simulink model "snap2_f_200msps_64i_4096c"  (R2019a)
settings: Solver=VariableStepDiscrete  StartTime=0.0  StopTime=10.0  RelTol=1e-3
undefined symbols (not defined in the file or in its folder): datetime, posixtime
libraries: xbsIndex_r4 x21354, casper_library_misc x297, casper_library_delays x19, xps_library x14, casper_library_sources x4
(part 1 of 217)
settings Model: ModifiedComment=jackh -- Fri May 23 06:17:14 2025 -- Version 1.665  Creator=mdexter  LastModifiedBy=jackh
settings Model: ModifiedHistory=|
  | jackh -- Fri May 23 06:17:14 2025 -- Version 1.665
  | 
  | jackh -- Thu May 22 05:48:14 2025 -- Version 1.664
  | 
  | v7.4.0.0 -- Expand number of coefficients to one per channel
  | 
  | kplant -- Fri Aug 11 09:07:04 2023 -- Version 1.663
  | Saving after compiling
  | 
  | kplant -- Thu Aug 10 22:12:33 2023 -- Version 1.662
  | Version 7.3.2.1 now has pipelines with a latency of 3 before the f-engine's ethernet block.
  | 
  | kplant -- Thu Aug 10 10:59:50 2023 -- Version 1.661
  | Version 7.3.2.0 increases the pipeline latency to 2 in front of the f-engine 40Gbe block and changes the target clock rate to 196 MHz.
  | 
  | kplant -- Wed Aug 09 13:06:15 2023 -- Version 1.660
  | Added pipeline blocks with a latency of 1 before each of the inputs to the 40Gb ethernet block that the f-engine uses.
  | 
  | kplant -- Tue Aug 08 14:00:49 2023 -- Version 1.659
  | 
  | kplant -- Tue Aug 08 13:55:20 2023 -- Version 1.658
  | Adding cosmic ray system version 6.0.1.0 which has the FIR and so far has only been compiled from snap2_f_200msps_64i_4096c_nopfb.slx
  | 
  | kplant -- Thu Apr 27 20:02:10 2023 -- Version 1.657
  | Saving after compile.
  | 
  | kplant -- Wed Apr 26 17:00:51 2023 -- Version 1.656
  | I removed the delay trigger option and changed it to an option to delay the input to the buffer, in order to be able to position the pulse in the center of the buffer.
  | 
  | kplant -- Fri Apr 07 12:31:25 2023 -- Version 1.655
  | Add cosmic ray version 5.0.0.1 and change main version to 7.3.0.2.
  | 
  | kplant -- Thu Apr 06 14:32:58 2023 -- Version 1.654
  | Saving after compiling 7.3.0.1.
  | 
  | jackh -- Thu Apr 06 12:53:56 2023 -- Version 1.653
  | 
  | Make CR block and mask block use sync_time, not telescope_time
  | 
  | kplant -- Fri Mar 24 06:24:14 2023 -- Version 1.652
  | Saving after compiling version 7.3 with cosmic ray system 5.0.0.
  | 
  | jackh -- Wed Mar 08 22:10:30 2023 -- Version 1.651
  | 
  | compiled
  | 
  | jackh -- Wed Mar 08 15:15:31 2023 -- Version 1.650
  | rev 7.2
  | 2 bits below EQ binary point
  | 
  | jackh -- Thu Feb 16 17:13:47 2023 -- Version 1.649
  | 
  | compiled
  | 
  | jackh -- Thu Feb 16 09:43:58 2023 -- Version 1.648
  | 
  | Remove hard-coded first 5-stages of shift
  | 
  | jackh -- Wed Feb 15 17:04:22 2023 -- Version 1.647
  | 
  | compiled
  | 
  | jackh -- Tue Feb 14 18:32:23 2023 -- Version 1.646
  | 
  | Change EQ fractional bits from 5 to 4
  | Rebuild FFT IP with all serial stages optional shift
  | 
  | jackh -- Thu Jan 05 10:26:17 2023 -- Version 1.645
  | v7.0.0 as compiled
  | 
  | jackh -- Wed Jan 04 19:36:26 2023 -- Version 1.644
  | 
  | jackh -- Wed Jan 04 19:34:58 2023 -- Version 1.643
  | v7.0.0.0
  | CR version 4.3.1
  | 
  | jackh -- Tue Dec 20 11:37:43 2022 -- Version 1.642
  | 
  | compiled 6.1. 4 x 0.003ns timing errors, only on unused CR 40GbE RX path.
  | 
  | 
  | jackh -- Fri Dec 16 15:06:04 2022 -- Version 1.641
  | 
  | jackh -- Fri Dec 16 14:46:34 2022 -- Version 1.640
  | 
  | jackh -- Fri Dec 16 14:13:03 2022 -- Version 1.639
  | 
  | jackh -- Fri Dec 16 13:41:06 2022 -- Version 1.638
  | 
  | 6.1 -- add per-signal flag threshold
  | 
  | jackh -- Fri Dec 16 11:47:24 2022 -- Version 1.637
  | 
  | jackh -- Fri Dec 16 11:47:00 2022 -- Version 1.636
  | 
  | jackh -- Thu Dec 15 20:54:27 2022 -- Version 1.635
  | 
  | Add acc_time registers
  | 
  | jackh -- Thu Dec 15 12:49:42 2022 -- Version 1.634
  | 
  | Include all 4 mask cores (whoops!)
  | 
  | jackh -- Thu Dec 15 12:39:59 2022 -- Version 1.633
  | 
  | Change max coarse delay to 4096 (previous compile didn't meet timing)
  | 
  | jackh -- Wed Dec 14 18:27:06 2022 -- Version 1.632
  | 
  | Add "mask" block, which allows zero-ing out spectra
  | whose total power exceed a runtime-controllable
  | threshold
  | 
  | kplant -- Wed Jun 01 13:17:05 2022 -- Version 1.631
  | 
  | kplant -- Wed Jun 01 07:18:09 2022 -- Version 1.630
  | 
  | kplant -- Wed Jun 01 06:41:48 2022 -- Version 1.629
  | Fixed telescope time input to cosmic ray block.
  | 
  | kplant -- Wed Jun 01 06:39:11 2022 -- Version 1.628
  | Commented out scopes
  | 
  | kplant -- Tue May 31 12:58:33 2022 -- Version 1.627
  | Cosmic ray version 4.1. Takes in telescope time, attempts to fix bug where trigger signal is blocked from starting packetizer.
  | 
  | kplant -- Tue May 31 12:56:22 2022 -- Version 1.626
  | 
  | kplant -- Tue May 31 09:44:09 2022 -- Version 1.625
  | 
  | jackh -- Fri May 13 14:05:09 2022 -- Version 1.624
  | 
  | Compiled 5.1.1.0 (CR rev 4)
  | 
  | jackh -- Thu May 12 12:01:29 2022 -- Version 1.623
  | 
  | Add PPS count register (which software already assumes exists!)
  | 
  | jackh -- Thu May 12 11:34:03 2022 -- Version 1.622
  | 
  | v5.1.0
  | Manual merge in of v4.0 CR module
  | 
  | jackh -- Thu Apr 14 04:49:04 2022 -- Version 1.621
  | 
  | jackh -- Wed Mar 23 12:35:09 2022 -- Version 1.620
  | 
  | Manually merce cosmic_ray_system.slx into the cosmic_ray subsystem
  | of this model. cosmic_ray_system appears to be version 3 (based on version register).
  | 
  | Bump main model version to 5.0.0.0
  | 
  | jackh -- Tue Jan 11 12:36:06 2022 -- Version 1.619
  | 
  | jackh -- Mon Jan 10 21:45:35 2022 -- Version 1.618
  | 
  | Bump bugfix
  | 
  | jackh -- Mon Jan 10 21:43:35 2022 -- Version 1.617
  | 
  | jackh -- Mon Jan 10 21:39:42 2022 -- Version 1.616
  | 
  | jackh -- Mon Jan 10 21:33:55 2022 -- Version 1.615
  | 
  | jackh -- Mon Jan 10 21:16:30 2022 -- Version 1.614
  | 
  | Fix bit width of sum(sq(ADC value)) -- was configured for 8 bit ADCs!
  | 
  | jackh -- Mon Nov 15 21:56:57 2021 -- Version 1.613
  | 
  | compiled
  | 
  | jackh -- Mon Nov 15 11:54:45 2021 -- Version 1.612
  | 
  | v4.6.0 -- add internal loopback for sync logic
  | 
  | jackh -- Fri Sep 17 19:23:29 2021 -- Version 1.611
  | 
  | Compiled with clean timing
  | 
  | 
  | jackh -- Fri Sep 17 13:13:59 2021 -- Version 1.610
  | 4.5.4 CR update
  | 
  | jackh -- Tue Sep 14 19:01:48 2021 -- Version 1.609
  | 
  | jackh -- Tue Sep 14 10:37:44 2021 -- Version 1.608
  | 
  | Change CR buffer BRAMs to have latency 2 and optimize for speed.
  | 
  | jackh -- Mon Sep 13 20:49:56 2021 -- Version 1.607
  | 
  | jackh -- Mon Sep 13 20:30:25 2021 -- Version 1.606
  | 
  | 4.5.3
  | Increase latency of autocorr vacc adders to 4
  | Change CR veto pulse extend subtract-1 to implement behaviourally
  | 
  | jackh -- Mon Sep 13 20:29:50 2021 -- Version 1.605
  | 
  | jackh -- Mon Sep 13 10:57:29 2021 -- Version 1.604
  | 
  | v4.5.2
  | 
  | Update CR subsys. Not sure whether this has actually changed,
  | but there was a commit to the repo. Using 14655219acb09ca
  | 
  | jackh -- Mon Sep 13 10:51:07 2021 -- Version 1.603
  | 
  | jackh -- Sun Sep 12 12:08:30 2021 -- Version 1.602
  | 
  | 4.5.1 -- update CR subsys
  | 
  | jackh -- Tue Aug 31 13:12:34 2021 -- Version 1.601
  | 
  | jackh -- Wed Aug 25 19:11:33 2021 -- Version 1.600
  | 
  | jackh -- Tue Aug 24 13:10:24 2021 -- Version 1.599
  | 
  | Fix delay readout bug
  | 
  | jackh -- Tue Aug 24 12:10:39 2021 -- Version 1.598
  | 
  | compiled. Missed timing, but only on 40G RX paths and within the 200MHz->196MHz margin
  | 
  | jackh -- Mon Aug 23 18:54:36 2021 -- Version 1.597
  | 
  | update CR
  | 
  | jackh -- Mon Aug 23 18:52:51 2021 -- Version 1.596
  | 
  | compiled
  | 
  | jackh -- Mon Aug 16 15:01:28 2021 -- Version 1.595
  | 
  | re-fix delay readout
  | 
  | jackh -- Mon Aug 16 14:36:11 2021 -- Version 1.594
  | 
  | compiled v4.3.0
  | 
  | jackh -- Fri Aug 13 12:33:00 2021 -- Version 1.593
  | 
  | jackh -- Fri Aug 13 12:32:21 2021 -- Version 1.592
  | 
  | jackh -- Fri Aug 13 12:30:04 2021 -- Version 1.591
  | 
  | Make autocorr vacc all float32
  | 
  | jackh -- Fri Aug 13 12:16:09 2021 -- Version 1.590
  | 
  | jackh -- Fri Aug 13 12:09:57 2021 -- Version 1.589
  | 
  | jackh -- Thu Aug 12 18:59:45 2021 -- Version 1.588
  | 
  | jackh -- Thu Aug 12 10:15:56 2021 -- Version 1.587
  | 
  | Remove CR 40GbE TX snapshot
  | 
  | jackh -- Thu Aug 12 10:13:47 2021 -- Version 1.586
  | 
  | Misc pipelining
  | 
  | jackh -- Wed Aug 11 12:31:06 2021 -- Version 1.585
  | 
  | jackh -- Wed Aug 11 12:26:16 2021 -- Version 1.584
  | 
  | v4.4
  | 
  | jackh -- Wed Aug 11 12:25:20 2021 -- Version 1.583
  | 
  | Combine some software registers in CR subsys
  | Combine delay registers into a RAM to (try to) reduce wishbone interconnect
  | 
  | jackh -- Wed Aug 11 11:56:18 2021 -- Version 1.582
  | 
  | Change delay registering to store delays in bram
  | 
  | jackh -- Wed Aug 11 11:10:53 2021 -- Version 1.581
  | 
  | Reduce number of noise generators to 4.
  | Control noise fanout to multiplexers
  | 
  | jackh -- Tue Aug 10 11:27:32 2021 -- Version 1.580
  | 
  | jackh -- Tue Aug 10 11:26:01 2021 -- Version 1.579
  | 
  | fix EQ coefficient addressing
  | 
  | jackh -- Tue Aug 10 11:02:45 2021 -- Version 1.578
  | 
  | jackh -- Mon Aug 09 21:32:19 2021 -- Version 1.577
  | 
  | jackh -- Mon Aug 09 21:31:35 2021 -- Version 1.576
  | 
  | jackh -- Mon Aug 09 18:30:08 2021 -- Version 1.575
  | 
  | compiled
  | 
  | jackh -- Mon Aug 09 10:43:25 2021 -- Version 1.574
  | 
  | jackh -- Mon Aug 09 10:40:58 2021 -- Version 1.573
  | 
  | jackh -- Mon Aug 09 10:31:43 2021 -- Version 1.572
  | 
  | Add pipeline registers on high-fanout CR subsystem sw register outputs
  | 
  | jackh -- Sun Aug 08 14:34:28 2021 -- Version 1.571
  | 
  | v4.3.0
  | 
  | jackh -- Sun Aug 08 14:24:45 2021 -- Version 1.570
  | 
  | jackh -- Sun Aug 08 14:11:25 2021 -- Version 1.569
  | 
  | jackh -- Sun Aug 08 13:31:26 2021 -- Version 1.568
  | 
  | Go back to floating point autocorr. Previous design used more ram and failed timing
  | 
  | jackh -- Sat Aug 07 15:01:43 2021 -- Version 1.567
  | 
  | Change chan_reorder double buffers to optimize for area
  | (sometimes halves the number of brams)
  | 
  | jackh -- Sat Aug 07 14:54:24 2021 -- Version 1.566
  | 
  | v4.2.0
  | 
  | Make autocorr 64-bit fixed point (to save floating cast)
  | Remove serial reorder from FFT and make part of EQ.
  | Compensate by bitbashing addresses for autocorr readout and EQ coefficients
  | 
  | 
  | jackh -- Sat Aug 07 14:49:26 2021 -- Version 1.565
  | 
  | jackh -- Sat Aug 07 14:41:23 2021 -- Version 1.564
  | 
  | jackh -- Sat Aug 07 14:24:43 2021 -- Version 1.563
  | 
  | jackh -- Sat Aug 07 13:38:58 2021 -- Version 1.562
  | 
  | Try to optimize pre-PFB reorder buffers
  | 
  | jackh -- Sat Aug 07 13:18:16 2021 -- Version 1.561
  | 
  | jackh -- Sat Aug 07 13:16:02 2021 -- Version 1.560
  | 
  | Put back in clip count registers because LRD uses them
  | 
  | jackh -- Sat Aug 07 12:39:11 2021 -- Version 1.559
  | 
  | jackh -- Sat Aug 07 12:19:25 2021 -- Version 1.558
  | 
  | compiled. Missed timing on one path by 0.04ns
  | 
  | jackh -- Tue Aug 03 11:43:54 2021 -- Version 1.557
  | 
  | jackh -- Tue Aug 03 11:14:29 2021 -- Version 1.556
  | 
  | Fix double up of delay RAM
  | 
  | jackh -- Tue Aug 03 11:04:58 2021 -- Version 1.555
  | 
  | 4.2.1 -- put CR QSP on port 2
  | 
  | jackh -- Mon Aug 02 12:46:12 2021 -- Version 1.554
  | 
  | Remove RX-side debug counters in CR 40G core
  | 
  | jackh -- Mon Aug 02 12:36:50 2021 -- Version 1.553
  | 
  | Make input power calculation use DSP
  | Change some input delays to behavioural
  | Change delay block to implement a single delay
  | with programmable delay from 0 to 1023, followed by 7
  | fixed 1024 clock delays which may be optionally bypassed.
  | Hopefully this will use less power.
  | 
  | jackh -- Mon Aug 02 11:15:00 2021 -- Version 1.552
  | 
  | implementation optimizations in CR block
  | 
  | jackh -- Mon Aug 02 10:53:02 2021 -- Version 1.551
  | 
  | jackh -- Sun Aug 01 12:01:07 2021 -- Version 1.550
  | make CR use LED 3 to prevent clash
  | 
  | jackh -- Sun Aug 01 10:17:04 2021 -- Version 1.549
  | 
  | v 4.1.0
  | uncomment CR.
  | 
  | jackh -- Sun Aug 01 10:02:19 2021 -- Version 1.548
  | 
  | jackh -- Sat Jul 31 15:41:04 2021 -- Version 1.547
  | v4.0.4 -- prep to compile with pre-placement power opt
  | 
  | jackh -- Sat Jul 31 11:19:09 2021 -- Version 1.546
  | 
  | jackh -- Fri Jul 30 17:49:37 2021 -- Version 1.545
  | 
  | jackh -- Fri Jul 30 17:45:17 2021 -- Version 1.544
  | 
  | rev 4.0.3
  | 
  | jackh -- Fri Jul 30 17:36:17 2021 -- Version 1.543
  | 
  | make autocorr float cast latency 4 again (failed timing)
  | set all map latencies on pre-pfb reorder to 2 (failed timing)
  | 
  | Copy all pfb cores so they match. A bug was introduced where core 0
  | had a 1 cycle latency difference to the others
  | 
  | jackh -- Fri Jul 30 12:38:28 2021 -- Version 1.542
  | 
  | shared bram latency to 1 in corr block
  | 
  | jackh -- Fri Jul 30 12:37:15 2021 -- Version 1.541
  | 
  | reduce shared bram latency to 1 in eqtvg
  | 
  | jackh -- Fri Jul 30 12:35:00 2021 -- Version 1.540
  | 
  | Reduce shared bram latency to 1 in autocorr and EQ blocks
  | 
  | jackh -- Fri Jul 30 12:31:43 2021 -- Version 1.539
  | 
  | Add option to tie autocorr data inputs to zero (to save a little power)
  | Reduce autocorr mux input latency 2->1
  | Reduce autocorr floating point cast latency 4->3
  | 
  | jackh -- Fri Jul 30 11:48:33 2021 -- Version 1.538
  | 
  | 4.0.2
  | Optimize bram delays for power
  | 
  | jackh -- Fri Jul 30 11:45:47 2021 -- Version 1.537
  | 
  | compiled
  | 
  | jackh -- Thu Jul 29 17:56:15 2021 -- Version 1.536
  | 
  | 4.0.1
  | 
  | Make a couple of brams optimize for power. Rebuild FFT / FIR to use (hopefully) less logic.
  | 
  | jackh -- Tue Jul 27 18:46:01 2021 -- Version 1.535
  | 
  | jackh -- Tue Jul 27 16:53:09 2021 -- Version 1.534
  | 
  | add in CR firmware (but comment out)
  | bump version to 4.0.0
  | 
  | 
  | jackh -- Tue Jul 27 16:23:54 2021 -- Version 1.533
  | 
  | jackh -- Tue Jul 27 16:22:45 2021 -- Version 1.532
  | 
  | Make 4-bit quantize use DSP core. Remove 4-bit clip count. it's basically useless unless broken down by freq channel
  | 
  | jackh -- Tue Jul 27 16:11:15 2021 -- Version 1.531
  | 
  | jackh -- Tue Jul 27 10:57:43 2021 -- Version 1.530
  | 
  | as compiled
  | 
  | jackh -- Mon Jul 26 20:52:28 2021 -- Version 1.529
  | 
  | jackh -- Mon Jul 26 20:39:42 2021 -- Version 1.528
  | 
  | jackh -- Mon Jul 26 14:40:36 2021 -- Version 1.527
  | 
  | Add IODELAYs on timing signals. Add ext PPS variations register
  | 
  | 
  | jackh -- Mon Jul 26 13:07:19 2021 -- Version 1.526
  | 
  | jackh -- Mon Jul 26 13:02:55 2021 -- Version 1.525
  | 
  | jackh -- Mon Jul 26 12:04:41 2021 -- Version 1.524
  | 
  | jackh -- Fri Jul 23 16:52:58 2021 -- Version 1.523
  | 
  | jackh -- Fri Jul 23 16:41:18 2021 -- Version 1.522
  | 
  | jackh -- Thu Jul 22 17:52:28 2021 -- Version 1.521
  | 
  | jackh -- Thu Jul 22 12:41:40 2021 -- Version 1.520
  | 
  | jackh -- Thu Jul 22 12:33:28 2021 -- Version 1.519
  | 
  | jackh -- Thu Jul 22 12:03:06 2021 -- Version 1.518
  | 
  | jackh -- Thu Jul 22 12:02:39 2021 -- Version 1.517
  | 
  | jackh -- Thu Jul 22 11:51:17 2021 -- Version 1.516
  | 
  | rev 3.4
  | 
  | jackh -- Thu Jul 22 11:33:52 2021 -- Version 1.515
  | 
  | Add trigger logic to autocorr spectrum grabbing
  | 
  | jackh -- Wed Jul 14 19:19:47 2021 -- Version 1.514
  | 
  | Bump version to 3.3.0
  | 
  | jackh -- Wed Jul 14 19:18:36 2021 -- Version 1.513
  | 
  | Add PFB FIR bypass
  | 
  | 
  | jackh -- Tue Jul 06 15:20:17 2021 -- Version 1.512
  | 
  | jackh -- Thu Jul 01 15:44:46 2021 -- Version 1.511
  | 
  | jackh -- Thu Jul 01 15:41:36 2021 -- Version 1.510
  | 
  | jackh -- Thu Jul 01 15:38:13 2021 -- Version 1.509
  | 
  | Bump version to 3.2.1
  | 
  | jackh -- Thu Jul 01 14:31:27 2021 -- Version 1.508
  | 
  | Add enable to ADC external chip sync
  | 
  | jackh -- Thu Jul 01 12:43:11 2021 -- Version 1.507
  | as compiled
  | 
  | jackh -- Wed Jun 30 19:07:36 2021 -- Version 1.506
  | 
  | jackh -- Wed Jun 30 19:06:42 2021 -- Version 1.505
  | 
  | Bugfix 1 -- double-buffered reorders seem broken?!
  | 
  | jackh -- Tue Jun 29 18:31:06 2021 -- Version 1.504
  | 
  | jackh -- Tue Jun 29 18:30:15 2021 -- Version 1.503
  | 
  | jackh -- Tue Jun 29 14:35:01 2021 -- Version 1.502
  | 
  | Add PPS period counter.
  | Extend output sync pulse to 1024 clocks
  | 
  | jackh -- Thu Jun 17 11:51:33 2021 -- Version 1.501
  | 
  | jackh -- Wed Jun 16 11:07:37 2021 -- Version 1.500
  | 
  | jackh -- Wed Jun 16 11:02:07 2021 -- Version 1.499
  | 
  | Bump version to 3.1.0
  | 
  | Add Zynq interfaces:
  |   - Power monitoring I2C
  |   - PPS GPIO input
  | 
  | Requires Zynq to be programmed with appropriate bitstream.
  | 
  | jackh -- Tue Jun 15 15:37:49 2021 -- Version 1.498
  | 
  | Change ADC versions to rev 2 (updated pinout)
  | Bump firmware version to 3.0.0
  | 
  | jackh -- Thu Jun 10 13:30:51 2021 -- Version 1.497
  | 
  | bugfix 3
  | 
  | Off-by-1 autocorr channel error
  | 
  | jackh -- Thu Jun 10 12:13:26 2021 -- Version 1.496
  | 
  | compile. Bump bugfix to 2
  | 
  | jackh -- Wed Jun 09 12:36:01 2021 -- Version 1.495
  | 
  | FFT of bit inversion fix
  | 
  | jackh -- Tue Jun 08 19:39:36 2021 -- Version 1.494
  | 
  | jackh -- Tue Jun 08 18:24:07 2021 -- Version 1.493
  | 
  | off-by-one integration bug in autocorr acc
  | 
  | jackh -- Fri May 14 17:02:59 2021 -- Version 1.492
  | 
  | Remove a pipeline register after the ADCs.
  | Trying to free up routing at the FIFO inputs to make the compiler's life easier.
  | 
  | jackh -- Fri May 14 09:09:53 2021 -- Version 1.491
  | 
  | as compiled
  | 
  | jackh -- Wed May 05 14:45:26 2021 -- Version 1.490
  | 
  | Version bump prior to recompiling with new ADC interface (with bitslip)
  | 
  | jackh -- Tue Apr 13 20:04:05 2021 -- Version 1.489
  | 
  | jackh -- Tue Apr 13 20:01:34 2021 -- Version 1.488
  | 
  | docstrings
  | 
  | jackh -- Tue Apr 13 19:38:13 2021 -- Version 1.487
  | 
  | updates OK
  | 
  | jackh -- Tue Apr 13 19:29:45 2021 -- Version 1.486
  | 
  | docstrings
  | 
  | jackh -- Tue Apr 13 19:14:40 2021 -- Version 1.485
  | 
  | docstrings in sync subsys
  | 
  | jackh -- Tue Apr 13 19:00:08 2021 -- Version 1.484
  | 
  | jackh -- Tue Apr 13 18:57:55 2021 -- Version 1.483
  | 
  | update 40G core with docstrings
  | 
  | 
  | jackh -- Tue Apr 13 18:42:31 2021 -- Version 1.482
  | 
  | jackh -- Tue Apr 13 18:20:50 2021 -- Version 1.481
  | 
  | docstrings
  | 
  | jackh -- Tue Apr 13 17:57:44 2021 -- Version 1.480
  | 
  | jackh -- Tue Apr 13 17:52:27 2021 -- Version 1.479
  | 
  | jackh -- Tue Apr 13 17:44:36 2021 -- Version 1.478
  | 
  | docstrings
  | 
  | jackh -- Tue Apr 13 17:36:01 2021 -- Version 1.477
  | 
  | docstrings
  | 
  | jackh -- Tue Apr 13 17:25:32 2021 -- Version 1.476
  | 
  | jackh -- Tue Apr 13 17:20:03 2021 -- Version 1.475
  | 
  | jackh -- Tue Apr 13 17:12:39 2021 -- Version 1.474
  | 
  | regenerate brams including autodocs
  | 
  | jackh -- Tue Apr 13 16:48:19 2021 -- Version 1.473
  | 
  | update software registers to include docstrings
  | 
  | jackh -- Tue Apr 13 16:04:09 2021 -- Version 1.472
  | 
  | jackh -- Tue Apr 13 10:32:10 2021 -- Version 1.471
  | 
  | Update software registers to include description field.
  | Step 1 in the grand plan to autodocument
  | 
  | jackh -- Thu Apr 08 11:57:43 2021 -- Version 1.470
  | 
  | Change FFT overflow registers to counters rather than flags
  | 
  | jackh -- Sun Mar 28 18:37:18 2021 -- Version 1.469
  | 
  | Misc timing internals pipelining
  | 
  | jackh -- Sun Mar 28 18:35:09 2021 -- Version 1.468
  | 
  | Unsurprisingly, a 64-bit DSP counter isn't allowed :)
  | Use HDL
  | 
  | jackh -- Sun Mar 28 18:29:55 2021 -- Version 1.467
  | 
  | Implement TT counter with DSP
  | 
  | jackh -- Sun Mar 28 18:28:20 2021 -- Version 1.466
  | 
  | rev up to 2.2.2
  | 
  | jackh -- Sun Mar 28 18:27:31 2021 -- Version 1.465
  | 
  | Add pipelining to sync_in GPIO
  | 
  | jackh -- Sun Mar 28 17:31:26 2021 -- Version 1.464
  | 
  | bump version to 2.2.1
  | 
  | jackh -- Sun Mar 28 17:20:11 2021 -- Version 1.463
  | 
  | jackh -- Sun Mar 28 17:17:29 2021 -- Version 1.462
  | 
  | Fix to spectra count latency in autocorrelation
  | 
  | jackh -- Sun Mar 28 16:47:41 2021 -- Version 1.461
  | 
  | Reduce max acc_len to 17 bits to match control register
  | 
  | jackh -- Sun Mar 28 16:04:04 2021 -- Version 1.460
  | 
  | jackh -- Sun Mar 28 10:30:48 2021 -- Version 1.459
  | 
  | 
  | 
  | jackh -- Sat Mar 27 16:35:07 2021 -- Version 1.458
  | 
  | jackh -- Sat Mar 27 16:33:52 2021 -- Version 1.457
  | 
  | jackh -- Sat Mar 27 16:33:04 2021 -- Version 1.456
  | 
  | Mux autocorrs to free up RAM. Prep to rebuild with interleaved PFB, which fell out the library
  | 
  | jackh -- Sat Mar 27 14:15:08 2021 -- Version 1.455
  | 
  | inconsequential block name changes in noise generator
  | 
  | jackh -- Sat Mar 27 14:01:25 2021 -- Version 1.454
  | 
  | remove posedges from ADC control signals
  | (some of these need to be registered into a domain with a clock half the rate of simulink)
  | 
  | jackh -- Fri Mar 19 15:12:44 2021 -- Version 1.453
  | 
  | jackh -- Tue Mar 16 12:34:32 2021 -- Version 1.452
  | 
  | Add internal ADC sync register. Bump version to 2.1.0
  | 
  | jackh -- Tue Mar 16 11:03:32 2021 -- Version 1.451
  | 
  | jackh -- Tue Mar 09 10:10:05 2021 -- Version 1.450
  | 
  | jackh -- Tue Mar 09 10:05:23 2021 -- Version 1.449
  | 
  | jackh -- Tue Mar 09 10:03:37 2021 -- Version 1.448
  | 
  | jackh -- Mon Mar 01 11:44:07 2021 -- Version 1.447
  | 
  | jackh -- Sun Feb 28 13:35:39 2021 -- Version 1.446
  | 
  | update clocks to use FMC1 (since that's the only prototype ADC board we can use)
  | 
  | jackh -- Sun Feb 28 13:26:05 2021 -- Version 1.445
  | 
  | Pipelining on ADC output; 40GbE input
  | 
  | jackh -- Sat Feb 27 12:53:30 2021 -- Version 1.444
  | 
  | jackh -- Fri Feb 26 19:07:36 2021 -- Version 1.443
  | 
  | jackh -- Fri Feb 26 19:03:07 2021 -- Version 1.442
  | 
  | Store autocorrs as 32-bit floats (to save RAM)
  | 
  | jackh -- Thu Feb 25 20:40:57 2021 -- Version 1.441
  | 
  | jackh -- Thu Feb 25 20:35:24 2021 -- Version 1.440
  | 
  | autocorr fixes
  | 
  | 
  | jackh -- Tue Feb 23 18:00:30 2021 -- Version 1.439
  | 
  | Add snapshot trigger to ADC(s)
  | 
  | jackh -- Tue Feb 23 16:55:19 2021 -- Version 1.438
  | 
  | jackh -- Tue Feb 23 16:44:18 2021 -- Version 1.437
  | 
  | Add unquantized autocorr module
  | 
  | jackh -- Tue Feb 02 19:39:04 2021 -- Version 1.436
  | 
  | add adc_sync output
  | 
  | jackh -- Mon Dec 07 12:03:10 2020 -- Version 1.435
  | 
  | update ADCs to rev2
  | 
  | jackh -- Thu Nov 19 12:32:34 2020 -- Version 1.434
  | 
  | Updates to 4-bit quantize for timing improvements (hopefully)
  | 
  | jackh -- Tue Nov 17 11:51:00 2020 -- Version 1.433
  | 
  | Add rev / bugfix fields to version.
  | Add timestamp register -- storing UNIX timestamp of build (or, strictly, of last update time, I think)
  | 
  | 
  | jackh -- Tue Aug 11 17:16:40 2020 -- Version 1.432
  | 
  | snap2 -> rev 2
  | 
  | jackh -- Tue Aug 11 17:13:54 2020 -- Version 1.431
  | 
  | compiled
  | 
  | jackh -- Tue Aug 11 10:34:36 2020 -- Version 1.430
  | 
  | sync subsystem cleanup.
  | Add sync_time to packet header
  | 
  | jackh -- Tue Jul 28 17:40:14 2020 -- Version 1.429
  | 
  | Make some blocks  with registers inside gold
  | 
  | jackh -- Tue Jun 16 16:41:05 2020 -- Version 1.428
  | 
  | jackh -- Mon Jun 15 10:48:06 2020 -- Version 1.427
  | 
  | jackh -- Fri Jun 12 12:44:37 2020 -- Version 1.426
  | 
  | add chan_block_index field to output headers.
  | 
  | This should allow compatibility with the bifrost UDP capture framework
  | 
  | jackh -- Thu Jun 11 12:01:09 2020 -- Version 1.425
  | 
  | Update SNAP2 MSSGE block (new version has choice of FMC0/1 clock sourcing and SNAP2 hardware version selection)
  | 
  | jackh -- Thu Jun 11 11:59:20 2020 -- Version 1.424
  | update ADC blocks for single-FMC versions. Add ADC sync and reset registers
  | 
  | jackh -- Thu Jun 11 11:55:51 2020 -- Version 1.423
  | 
  | jackh -- Thu Jun 11 11:54:30 2020 -- Version 1.422
  | 
  | default n_pols to 64
  | 
  | jackh -- Thu Jun 11 11:44:03 2020 -- Version 1.421
  | 
  | make dest port 16-bits
  | add n_pols header entry
  | 
  | jackh -- Thu Jun 11 11:17:26 2020 -- Version 1.420
  | 
  | extra reserved 32-bit header entry
  | 
  | jackh -- Thu Jun 11 11:14:09 2020 -- Version 1.419
  | 
  | Reorg packet header to include n_chans, magic number, and reserver 32-bits
  | 
  | jackh -- Sun May 10 22:08:41 2020 -- Version 1.418
  | 
  | Make destination port selection per-packet
  | 
  | jackh -- Sun May 10 19:32:52 2020 -- Version 1.417
  | 
  | update chan-reorder to reorder pols in ascending order
  | 
  | jackh -- Fri May 08 15:11:27 2020 -- Version 1.416
  | 
  | update input block with RMS timing fixes
  | 
  | jackh -- Fri May 08 15:10:21 2020 -- Version 1.415
  | 
  | jackh -- Tue May 05 13:29:10 2020 -- Version 1.414
  | 
  | jackh -- Fri May 01 15:26:24 2020 -- Version 1.413
  | 
  | Use sys_clk for testing
  | 
  | jackh -- Fri May 01 15:14:39 2020 -- Version 1.412
  | 
  | Rename 1Gbe core so it is alphabetically first
  | 
  | jackh -- Fri May 01 15:11:49 2020 -- Version 1.411
  | 
  | jackh -- Fri May 01 11:15:12 2020 -- Version 1.410
  | 
  | Change 40gbe core enable so that software enable state can only change immediately after an EOF
  | 
  | jackh -- Fri Apr 24 17:52:32 2020 -- Version 1.409
  | 
  | jackh -- Fri Apr 24 17:51:51 2020 -- Version 1.408
  | 
  | jackh -- Fri Apr 24 17:50:48 2020 -- Version 1.407
  | 
  | jackh -- Fri Apr 24 17:48:49 2020 -- Version 1.406
  | 
  | make packetizer simpler
  | 
  | jackh -- Fri Apr 24 16:17:31 2020 -- Version 1.405
  | 
  | ass max_delay register to delay core
  | 
  | jackh -- Fri Apr 24 16:14:09 2020 -- Version 1.404
  | 
  | jackh -- Fri Apr 24 16:12:03 2020 -- Version 1.403
  | 
  | update eq_tvg to single bram
  | 
  | jackh -- Fri Apr 24 16:08:40 2020 -- Version 1.402
  | 
  | jackh -- Thu Apr 09 09:24:59 2020 -- Version 1.401
  | 
  | make delays 8k long
  | 
  | jackh -- Mon Mar 30 21:41:54 2020 -- Version 1.400
  | 
  | add 1gbe core
  | 
  | jackh -- Sat Mar 14 14:05:43 2020 -- Version 1.399
  | 
  | jackh -- Wed Feb 19 18:48:51 2020 -- Version 1.398
  | 
  | jackh -- Wed Feb 19 18:31:56 2020 -- Version 1.397
  | 
  | jackh -- Wed Feb 19 18:25:06 2020 -- Version 1.396
  | 
  | jackh -- Wed Feb 19 17:10:23 2020 -- Version 1.395
  | 
  | add back in reorders in pfb (having fixed mlib_devel)
  | 
  | jackh -- Tue Feb 18 17:39:49 2020 -- Version 1.394
  | 
  | 10 bitify
  | 
  | jackh -- Tue Feb 18 17:31:23 2020 -- Version 1.393
  | 
  | update_casper_blocks
  | 
  | jackh -- Fri Jan 24 08:04:16 2020 -- Version 1.392
  | replace ADC with sw regs to try and compile for SNAP2
  | 
  | jackh -- Wed Jan 08 08:41:40 2020 -- Version 1.391
  | 
  | 
  | jackh -- Wed Jan 08 08:26:20 2020 -- Version 1.390
  | 
  | 
  | jackh -- Wed Jan 08 08:24:50 2020 -- Version 1.389
  | 
  | 
  | jackh -- Wed Jan 08 08:23:40 2020 -- Version 1.388
  | 
  | 
  | jackh -- Wed Jan 08 08:22:29 2020 -- Version 1.387
  | update platform to SNAP2
  | 
  | jackh -- Wed Jan 08 08:21:36 2020 -- Version 1.386
  | 
  | 
  | jackh -- Wed Jan 08 08:21:09 2020 -- Version 1.385
  | Update internal cross-corr block
  | 
  | jackh -- Wed Jan 08 07:50:59 2020 -- Version 1.384
  | 
  | 
  | jackh -- Wed Jan 08 07:48:46 2020 -- Version 1.383
  | 
  | 
  | jackh -- Wed Jan 08 07:45:47 2020 -- Version 1.382
  | 
  | 
  | jackh -- Wed Jan 08 07:44:03 2020 -- Version 1.381
  | 
  | 
  | jackh -- Wed Jan 08 07:41:17 2020 -- Version 1.380
  | 
  | 
  | jackh -- Wed Jan 08 07:35:58 2020 -- Version 1.379
  | 
  | 
  | jackh -- Wed Jan 08 07:33:51 2020 -- Version 1.378
  | 
  | 
  | jackh -- Wed Jan 08 07:29:30 2020 -- Version 1.377
  | 
  | 
  | jackh -- Wed Jan 08 07:24:27 2020 -- Version 1.376
  | 1st pass fuilly updated to LWA spec
  | 
  | jackh -- Tue Jan 07 10:50:49 2020 -- Version 1.375
  | 
  | 
  | jackh -- Tue Jan 07 10:38:05 2020 -- Version 1.374
  | EQ tvg & FFT updated for 64 inputs
  | 
  | jackh -- Tue Jan 07 10:18:18 2020 -- Version 1.373
  | 
  | 
  | jackh -- Tue Jan 07 10:12:36 2020 -- Version 1.372
  | update FFT
  | 
  | jackh -- Tue Jan 07 09:22:52 2020 -- Version 1.371
  | update FFT core (currently only doing 1/4 of the necessary work)
  | 
  | jackh -- Tue Jan 07 07:40:39 2020 -- Version 1.370
  | Make 64-input. Only corrected up to FFT inputs
  | 
  | jackh -- Tue Jan 07 06:33:25 2020 -- Version 1.369
  | Save a version for LWA expansion project.
  | 
  | jackh -- Sun Oct 27 09:17:26 2019 -- Version 1.368
  | compiled
  | 
  | jackh -- Sun Oct 27 07:24:12 2019 -- Version 1.367
  | remove registering of reorder outputs
  | 
  | jackh -- Sun Oct 27 07:22:37 2019 -- Version 1.366
  | change input snapshot to snap only one of 3 inputs
  | 
  | jackh -- Sun Oct 27 03:59:18 2019 -- Version 1.365
  | remove some superfluous registers to improve timing.
  | Reduce snapshot in input block from 1k samples to 512
  | 
  | jackh -- Sun Oct 27 01:46:50 2019 -- Version 1.364
  | Fix FFT shift bitwidth bug
  | 
  | FFT core was expecting a 16-bit shift, but only a 12bit value was sliced from the control register
  | 
  | jackh -- Fri Aug 30 09:22:01 2019 -- Version 1.363
  | compiled
  | 
  | jackh -- Thu Aug 29 17:13:27 2019 -- Version 1.362
  | change delay shift reg to 3 bit addr
  | 
  | jackh -- Thu Aug 29 11:33:13 2019 -- Version 1.361
  | corr fixes
  | 
  | jackh -- Thu Aug 29 11:09:21 2019 -- Version 1.360
  | latency fix in eqtvg
  | 
  | jackh -- Thu Aug 29 10:02:04 2019 -- Version 1.359
  | compiled
  | 
  | jackh -- Wed Aug 28 15:31:00 2019 -- Version 1.358
  | bump to version 1.3
  | 
  | jackh -- Wed Aug 28 15:26:18 2019 -- Version 1.357
  | change quantization to saturate.
  | Change coefficients to 16_5 (was 16_6)
  | 
  | jackh -- Wed Aug 28 14:17:28 2019 -- Version 1.356
  | remove debugging snapshots hidden in corr vaccs
  | 
  | jackh -- Fri Aug 23 15:01:55 2019 -- Version 1.355
  | compiled
  | 
  | jackh -- Fri Aug 23 10:43:05 2019 -- Version 1.354
  | add snapshot in input block
  | 
  | jackh -- Thu Aug 22 17:13:50 2019 -- Version 1.353
  | fix to eqtvg ram depths
  | 
  | jackh -- Thu Aug 22 15:23:14 2019 -- Version 1.352
  | bump version to 1.2
  | 
  | jackh -- Thu Aug 22 15:22:39 2019 -- Version 1.351
  | Force pairs of pols to have same random number generator to save resources
  | 
  | jackh -- Thu Aug 22 15:19:21 2019 -- Version 1.350
  | rotator channel index counter fixes
  | 
  | eq tvg split bram into 3 (so we can have 6 channels, not 8)
  | 
  | jackh -- Thu Aug 22 12:01:44 2019 -- Version 1.349
  | 
  | 
  | jackh -- Thu Aug 22 12:01:21 2019 -- Version 1.348
  | Changes to rotator precision
  | 
  | jackh -- Tue Aug 20 19:46:09 2019 -- Version 1.347
  | compiled
  | 
  | jackh -- Tue Aug 20 16:55:38 2019 -- Version 1.346
  | increase minimum walsh period to 2**18 fpga clocks (was 2**13)
  | 
  | jackh -- Tue Aug 20 16:40:34 2019 -- Version 1.345
  | 
  | 
  | jackh -- Tue Aug 20 16:15:18 2019 -- Version 1.344
  | bump version to 1.1
  | 
  | jackh -- Tue Aug 20 16:14:49 2019 -- Version 1.343
  | add global enables to phase switch mod/demod to make software easier
  | 
  | jackh -- Mon Aug 19 17:54:23 2019 -- Version 1.342
  | compiled
  | 
  | jackh -- Thu Aug 01 11:53:22 2019 -- Version 1.341
  | make programmable sync delay tolerate delay=0
  | 
  | jackh -- Wed Jul 31 13:49:54 2019 -- Version 1.340
  | comment out corr->rms
  | 
  | jackh -- Mon Jul 29 17:05:34 2019 -- Version 1.339
  | delete corr rms block (not currently enough ram)
  | 
  | jackh -- Mon Jul 29 17:03:29 2019 -- Version 1.338
  | Add version block
  | 
  | jackh -- Mon Jul 29 16:58:22 2019 -- Version 1.337
  | make sync in have a programmable delay
  | Solves 2 problems:
  | 
  | 1) Can start integrations at arbitrary times (good for LST alignment)
  | 2) Can start a 16 second integration chunk on an arbitrary time boundary (needed to avoid the downstream correlator having 16 second start / stop granularity)
  | 
  | jackh -- Mon Jul 29 16:50:03 2019 -- Version 1.336
  | update phasor to 24-bits
  | 
  | jackh -- Sat May 11 17:48:41 2019 -- Version 1.335
  | 
  | 
  | jackh -- Sat May 11 17:46:07 2019 -- Version 1.334
  | 
  | 
  | jackh -- Sat May 11 17:45:44 2019 -- Version 1.333
  | 
  | 
  | jackh -- Sat May 11 17:40:04 2019 -- Version 1.332
  | 
  | 
  | jackh -- Sat May 11 17:36:59 2019 -- Version 1.331
  | add vacc for autocorrs @ 16 bit resolution
  | 
  | deepthi -- Sun Oct 28 15:16:19 2018 -- Version 1.330
  | 
  | 
  | deepthi -- Sat Oct 27 18:45:54 2018 -- Version 1.329
  | 
  | packetizer: Added an 'and' block that holds new_packet signal in high until the first sync.
  | 
  | deepthi -- Sat Oct 27 17:33:32 2018 -- Version 1.328
  | 
  | 1. Change edge_detect location in sync block
  | 
  | deepthi -- Sat Oct 20 22:13:43 2018 -- Version 1.327
  | 
  | 1. Add edge detect to software reg and gpio input in sync block.
  | 
  | 2. Add new corr block with max hold functionality.
  | 
  | jackh -- Tue Oct 09 20:34:13 2018 -- Version 1.326
  | recompile with pmbus_alert register
  | 
  | jackh -- Thu Jul 12 10:55:28 2018 -- Version 1.325
  | 
  | 
  | jackh -- Wed Jul 11 17:20:51 2018 -- Version 1.324
  | syntax
  | 
  | jackh -- Wed Jul 11 17:16:24 2018 -- Version 1.323
  | increase resolution of phase rotator bram.
  | 
  | jackh -- Wed Jul 11 17:10:41 2018 -- Version 1.322
  | 
  | 
  | jackh -- Tue Jul 10 16:08:30 2018 -- Version 1.321
  | scramble rotator channel multiplers to match PFB output order (hopefully)
  | 
  | jackh -- Tue Jul 10 15:51:56 2018 -- Version 1.320
  | 
  | 
  | jackh -- Tue Jul 10 13:37:24 2018 -- Version 1.319
  | fix off-by-one in slicing of mcnt counter, which was having the effect of duplicating mcnts in headers
  | 
  | jackh -- Sat Jul 07 14:17:05 2018 -- Version 1.318
  | compiled
  | 
  | jackh -- Fri Jul 06 10:33:47 2018 -- Version 1.317
  | fix bitbashing to rotator phase addresses
  | 
  | jackh -- Fri Jul 06 10:17:15 2018 -- Version 1.316
  | Add mux to enable / disable rotator
  | 
  | jackh -- Thu Jul 05 17:21:10 2018 -- Version 1.315
  | make some delays behavioural
  | 
  | jackh -- Thu Jul 05 14:48:28 2018 -- Version 1.314
  | 
  | 
  | jackh -- Thu Jul 05 14:46:13 2018 -- Version 1.313
  | 
  | 
  | jackh -- Thu Jul 05 14:43:36 2018 -- Version 1.312
  | 
  | 
  | jackh -- Thu Jul 05 14:40:00 2018 -- Version 1.311
  | 
  | 
  | jackh -- Thu Jul 05 14:36:19 2018 -- Version 1.310
  | 
  | 
  | jackh -- Thu Jul 05 14:26:16 2018 -- Version 1.309
  | integrate rotator into pipeline
  | 
  | jackh -- Thu Jul 05 14:20:20 2018 -- Version 1.308
  | 
  | create phase-rotation block
  | 
  | deepthi -- Thu Jun 07 09:24:03 2018 -- Version 1.307
  | 
  | Replaced the corr block.
  | 
  | deepthi -- Wed Jun 06 12:07:26 2018 -- Version 1.306
  | 
  | 
  | deepthi -- Tue Jun 05 17:46:17 2018 -- Version 1.305
  | 
  | Replaced the corr block with the tested version
  | 
  | deepthi -- Sat May 12 19:11:02 2018 -- Version 1.304
  | 
  | Changed time counter to increment between even/odd banks
  | 
  | deepthi -- Sat May 12 19:06:34 2018 -- Version 1.303
  | 
  | changed timing of eof, valid, data and headers
  | 
  | deepthi -- Mon May 07 23:03:07 2018 -- Version 1.302
  | 
  | 
  | deepthi -- Mon May 07 00:31:44 2018 -- Version 1.301
  | 
  | 
  | deepthi -- Fri May 04 20:13:43 2018 -- Version 1.300
  | 
  | Reduced width sliced from time_ctr
  | 
  | deepthi -- Fri May 04 19:47:57 2018 -- Version 1.299
  | 
  | Added delay to header and ip signals to account for pulse_ext on valid.
  | 
  | deepthi -- Fri May 04 19:23:23 2018 -- Version 1.298
  | 
  | 
  | deepthi -- Thu May 03 16:58:39 2018 -- Version 1.297
  | 
  | 1. Added delays to eof and dest_ip  to account for pulse_ext in valid.
  | 
  | 2. Changed eth_sw expected packet length to include header.
  | 
  | jackh -- Tue May 01 20:38:09 2018 -- Version 1.296
  | compiled
  | 
  | jackh -- Tue May 01 17:49:38 2018 -- Version 1.295
  | Fix to packetizer valid generation, to take into account the 3 (one per antenna) blocks of valid data in each stream of 512 channels
  | 
  | jackh -- Tue May 01 16:49:02 2018 -- Version 1.294
  | make channel selection bram 32-bits wide.
  | 
  | Remove GPU-packing mux / swreg
  | 
  | jackh -- Tue May 01 14:24:16 2018 -- Version 1.293
  | 
  | 
  | jackh -- Tue May 01 14:20:01 2018 -- Version 1.292
  | update chan reorderer
  | 
  | jackh -- Tue May 01 11:43:41 2018 -- Version 1.291
  | compiled
  | 
  | jackh -- Tue May 01 09:44:03 2018 -- Version 1.290
  | 
  | 
  | jackh -- Tue May 01 09:43:34 2018 -- Version 1.289
  | use bram for eq fft descramble map
  | 
  | jackh -- Tue May 01 09:40:26 2018 -- Version 1.288
  | change architecture of corr block -- now stores desired antennas in bram, rather than using a delay tree
  | 
  | jackh -- Mon Apr 30 20:21:35 2018 -- Version 1.287
  | 
  | 
  | jackh -- Mon Apr 30 20:18:20 2018 -- Version 1.286
  | 
  | 
  | jackh -- Mon Apr 30 20:15:51 2018 -- Version 1.285
  | compensate for FFT scrambling in EQ block. Descramble FFT post-requantization in this block
  | 
  | jackh -- Mon Apr 30 19:27:42 2018 -- Version 1.284
  | plausibility pass on corr block
  | 
  | jackh -- Mon Apr 30 12:16:47 2018 -- Version 1.283
  | 
  | 
  | jackh -- Mon Apr 30 12:14:25 2018 -- Version 1.282
  | store chan_reorder reorder map in bram
  | 
  | jackh -- Mon Apr 30 12:05:02 2018 -- Version 1.281
  | remove per-antenna histograms -- now get one histogram with multiplexed input
  | 
  | jackh -- Sun Apr 29 15:50:16 2018 -- Version 1.280
  | 
  | 
  | jackh -- Sun Apr 29 15:37:38 2018 -- Version 1.279
  | 
  | 
  | jackh -- Sun Apr 29 15:27:38 2018 -- Version 1.278
  | First pass packetizer. Regenerate pfb with parameter for serial block inputs
  | 
  | jackh -- Sat Mar 03 12:52:57 2018 -- Version 1.277
  | 
  | 
  | jackh -- Sun Feb 25 12:27:48 2018 -- Version 1.276
  | add pre-pfb reorder
  | 
  | jackh -- Sat Feb 24 13:39:06 2018 -- Version 1.275
  | 
  | jackh -- Sat Feb 24 13:38:40 2018 -- Version 1.274
  | update pfb to 16 inputs
  | 
  | jackh -- Fri Feb 23 18:44:26 2018 -- Version 1.273
  | 
  | 
  | jackh -- Fri Feb 23 18:38:20 2018 -- Version 1.272
  | 
  | 
  | jackh -- Fri Feb 23 17:01:30 2018 -- Version 1.271
  | make fft 8 parallel input
  | 
  | jackh -- Sat Feb 10 13:53:12 2018 -- Version 1.270
  | 
  | 
  | jackh -- Sat Feb 10 13:50:10 2018 -- Version 1.269
  | 
  | 
  | jackh -- Sat Feb 10 13:48:56 2018 -- Version 1.268
  | remove fft preshift
  | 
  | jackh -- Sat Feb 10 13:47:39 2018 -- Version 1.267
  | 
  | 
  | jackh -- Sat Feb 10 13:44:29 2018 -- Version 1.266
  | 
  | 
  | jackh -- Sat Feb 10 13:43:22 2018 -- Version 1.265
  | make delayer dual-pol
  | 
  | jackh -- Sat Feb 10 13:40:59 2018 -- Version 1.264
  | first pass new packet format with no time-based corner turn
  | 
  | jackh -- Fri Feb 09 17:29:05 2018 -- Version 1.263
  | 
  | 
  | jackh -- Fri Feb 09 15:23:03 2018 -- Version 1.262
  | first pass turning everything to 8192 channels
  | 
  | Changed the ants addr to be driven by the same signal that drives chans, ips (used to be driven by ant_tracker).
  | 
  | Removed nants software register that was previously thought to control time stamps (but didn't really)
  | 
  | deepthi -- Wed Jan 31 18:20:45 2018 -- Version 1.261
  | 
  | deepthi -- Mon Jan 29 17:20:36 2018 -- Version 1.260
  | 
  | 
  | deepthi -- Mon Jan 29 17:18:54 2018 -- Version 1.259
  | 
  | 
  | deepthi -- Mon Jan 29 17:18:33 2018 -- Version 1.258
  | 
  | 
  | deepthi -- Mon Jan 29 16:51:19 2018 -- Version 1.257
  | 
  | 
  | deepthi -- Mon Jan 29 16:46:46 2018 -- Version 1.256
  | 
  | 
  | deepthi -- Mon Jan 29 16:37:32 2018 -- Version 1.255
  | 
  | 
  | deepthi -- Mon Jan 29 16:11:03 2018 -- Version 1.254
  | 
  | 
  | deepthi -- Mon Jan 29 15:55:33 2018 -- Version 1.253
  | 
  | 
  | jackh -- Fri Nov 17 19:04:05 2017 -- Version 1.252
  | compiled
  | 
  | jackh -- Wed Nov 15 11:31:03 2017 -- Version 1.251
  | go to 3 corr blocks
  | 
  | jackh -- Tue Nov 14 16:10:40 2017 -- Version 1.250
  | 
  | 
  | jackh -- Tue Nov 14 15:28:37 2017 -- Version 1.249
  | reduce bram use in histogram shared brams
  | 
  | jackh -- Mon Nov 13 18:55:18 2017 -- Version 1.248
  | fix bug in histogram shared bram addr width
  | 
  | jackh -- Fri Nov 10 17:05:56 2017 -- Version 1.247
  | add 4 independent corr subsystems. Add EQ clipping counters
  | 
  | jackh -- Fri Nov 10 14:21:14 2017 -- Version 1.246
  | 
  | 
  | jackh -- Fri Nov 10 14:19:27 2017 -- Version 1.245
  | 
  | 
  | jackh -- Fri Nov 10 11:40:47 2017 -- Version 1.244
  | update to histograms v2
  | 
  | jackh -- Tue Nov 07 22:23:59 2017 -- Version 1.243
  | compiled -- passes eqtvg
  | 
  | jackh -- Tue Nov 07 20:41:00 2017 -- Version 1.242
  | 
  | 
  | jackh -- Tue Nov 07 20:39:30 2017 -- Version 1.241
  | packet header generation fixes
  | 
  | jackh -- Tue Nov 07 17:19:53 2017 -- Version 1.240
  | 
  | 
  | jackh -- Tue Nov 07 17:14:47 2017 -- Version 1.239
  | 
  | 
  | jackh -- Tue Nov 07 17:08:29 2017 -- Version 1.238
  | remove some chan_reorder debug snapshots
  | 
  | jackh -- Tue Nov 07 17:06:39 2017 -- Version 1.237
  | update ps GPIO pins
  | 
  | **** Change packetizer header blocks to can have a separate antenna / ip / chan for each packet. This is for the nants > 3 simulation modes. This will break previous versions of software *****
  | 
  | jackh -- Mon Nov 06 22:06:03 2017 -- Version 1.236
  | add comment to corr_acc_len
  | 
  | Compiled -- passes EQTVG test!
  | 
  | jackh -- Mon Nov 06 15:24:31 2017 -- Version 1.235
  | add OR block in mrst generator so that counter is enabled if/when an arm signal comes
  | 
  | jackh -- Sun Nov 05 21:39:25 2017 -- Version 1.234
  | comment on sync period
  | 
  | jackh -- Sun Nov 05 17:39:01 2017 -- Version 1.233
  | fix bitbasher in 32-spectra corner turn
  | 
  | jackh -- Sun Nov 05 17:05:17 2017 -- Version 1.232
  | aesthetic
  | 
  | jackh -- Sun Nov 05 17:02:53 2017 -- Version 1.231
  | changes to comments
  | 
  | jackh -- Sun Nov 05 17:01:27 2017 -- Version 1.230
  | make acc_len it's own register so we can acc to 2**32
  | 
  | jackh -- Sun Nov 05 16:58:57 2017 -- Version 1.229
  | 
  | 
  | jackh -- Sun Nov 05 16:56:52 2017 -- Version 1.228
  | add internal correlator
  | 
  | jackh -- Sun Nov 05 16:24:21 2017 -- Version 1.227
  | compiled.
  | 
  | jackh -- Sun Nov 05 15:19:13 2017 -- Version 1.226
  | latency tweak to data line in packetizer
  | 
  | jackh -- Sat Nov 04 20:21:54 2017 -- Version 1.225
  | change ethernet debug counters to 32 bits
  | 
  | jackh -- Sat Nov 04 20:05:10 2017 -- Version 1.224
  | make chan reorder map bram 32 bits to aid with software
  | 
  | jackh -- Sat Nov 04 19:51:25 2017 -- Version 1.223
  | change header brams to be 32-bit wide for all values.
  | This makes it easier to deal with the software, which can only write 32-bit bounded words.
  | 
  | jackh -- Sat Nov 04 14:23:39 2017 -- Version 1.222
  | replace big distributed ram in 16-spectra corner turn
  | with simple bit basher manipulation. The distributed ram tool a ridiculous amount of time to synthesize. Hopefully this will be faster.
  | 
  | jackh -- Fri Nov 03 16:25:40 2017 -- Version 1.221
  | 
  | 
  | jackh -- Fri Nov 03 16:17:13 2017 -- Version 1.220
  | update casper blocks on phase switch subsys
  | 
  | jackh -- Fri Nov 03 16:14:34 2017 -- Version 1.219
  | 
  | 
  | jackh -- Fri Nov 03 13:09:23 2017 -- Version 1.218
  | add phase switching and i2c control
  | 
  | jackh -- Fri Nov 03 12:43:29 2017 -- Version 1.217
  | 
  | add i2C controllers
  | 
  | jackh -- Mon Oct 23 16:15:14 2017 -- Version 1.216
  | Add back in Deepthi's fix from f3b63dae07d62
  | 
  | jackh -- Mon Oct 23 16:04:59 2017 -- Version 1.215
  | 
  | 
  | jackh -- Mon Oct 23 14:44:02 2017 -- Version 1.214
  | compiled. Still minor timing errors in the histograms
  | 
  | jackh -- Mon Oct 23 10:40:37 2017 -- Version 1.213
  | change EQ coeffs to one-per channel. Make format 16_6 (was 18_7)
  | 
  | jackh -- Mon Oct 09 15:00:17 2017 -- Version 1.212
  | 
  | halve number of brams in histogram readout
  | 
  | jackh -- Wed Sep 13 11:46:17 2017 -- Version 1.211
  | use built-in tge status regs
  | 
  | jackh -- Tue Sep 12 21:14:25 2017 -- Version 1.210
  | 
  | 
  | jackh -- Tue Sep 12 21:10:57 2017 -- Version 1.209
  | update_casper_blocks(bdroot)
  | 
  | jackh -- Tue Sep 12 21:02:11 2017 -- Version 1.208
  | add histogram to adc stats
  | 
  | jackh -- Fri Jul 14 11:30:38 2017 -- Version 1.207
  | set map = reord_map in chan_reorder blocks which use matlab scripts to generate their reorders.
  | 
  | jackh -- Thu Jul 13 17:48:05 2017 -- Version 1.206
  | change sync period to a 32-bit sw reg (was hardcoded 9! * 1024)
  | 
  | deepthi -- Thu Jul 13 13:07:36 2017 -- Version 1.205
  | 
  | 
  | deepthi -- Thu Jul 13 12:10:35 2017 -- Version 1.204
  | 
  | 
  | deepthi -- Wed Jul 12 16:52:46 2017 -- Version 1.203
  | 
  | 
  | deepthi -- Wed Jul 12 15:57:48 2017 -- Version 1.202
  | 
  | 
  | deepthi -- Tue Jul 11 19:00:41 2017 -- Version 1.201
  | 
  | 
  | deepthi -- Tue Jul 11 18:54:05 2017 -- Version 1.200
  | 
  | 
  | deepthi -- Tue Jul 11 18:52:32 2017 -- Version 1.199
  | 
  | 
  | deepthi -- Mon Jul 10 16:18:51 2017 -- Version 1.198
  | 
  | 
  | deepthi -- Sun Jul 09 18:15:02 2017 -- Version 1.197
  | 
  | 
  | deepthi -- Thu Jul 06 13:54:16 2017 -- Version 1.196
  | 
  | 
  | jackh -- Mon Jul 03 11:01:40 2017 -- Version 1.195
  | 
  | 
  | jackh -- Fri Jun 30 13:59:17 2017 -- Version 1.194
  | enable CPU tx/rx buffer on tge core. Needed for microblaze.
  | 
  | jackh -- Mon Jun 26 11:33:24 2017 -- Version 1.193
  | 
  | 
  | jackh -- Thu Jun 22 14:37:16 2017 -- Version 1.192
  | add history prompting
settings DataIOCC: LimitDataPoints=on  SaveFormat=Array  SignalLoggingSaveFormat=ModelDataLogs  ReturnWorkspaceOutputs=off
settings OptimizationCC: DefaultParameterBehavior=Inlined  ExpressionDepthLimit=2147483647  LifeSpan=inf
settings DebuggingCC: UnderspecifiedInitializationDetection=Classic  MergeDetectMultiDrivingBlocksExec=none  SolverPrmCheckMsg=warning  FcnCallInpInsideContextMsg=warning  AllowSymbolicDim=off  StateNameClashWarn=warning  SFUnexpectedBacktrackingDiag=warning  SFNoUnconditionalDefaultTransitionDiag=warning  SFExecutionAtInitializationDiag=none  ArithmeticOperatorsInVariantConditions=warning
settings HardwareCC: ProdBitPerPointer=32  ProdBitPerSizeT=32  ProdBitPerPtrDiffT=32  ProdLargestAtomicFloat=None  ProdIntDivRoundTo=Undefined  ProdEndianess=Unspecified  ProdWordSize=32  ProdHWDeviceType=32-bit Generic
settings ModelReferenceCC: PropagateSignalLabelsOutOfModel=off
settings SFSimCC: SimUseLocalCustomCode=off
settings RTWCC: RTWUseLocalCustomCode=off
settings CodeAppCC: StateflowObjectComments=on
settings GRTTargetCC: TargetLangStandard=C89/C90 (ANSI)  GeneratePreprocessorConditionals=Disable all  CombineOutputUpdateFcns=off  GRTInterface=on
settings ConfigComp: CovMetricSettings=dw  CovHtmlReporting=on  CovSaveCumulativeToWorkspaceVar=on  CovSaveSingleToWorkspaceVar=on  CovExternalEMLEnable=off

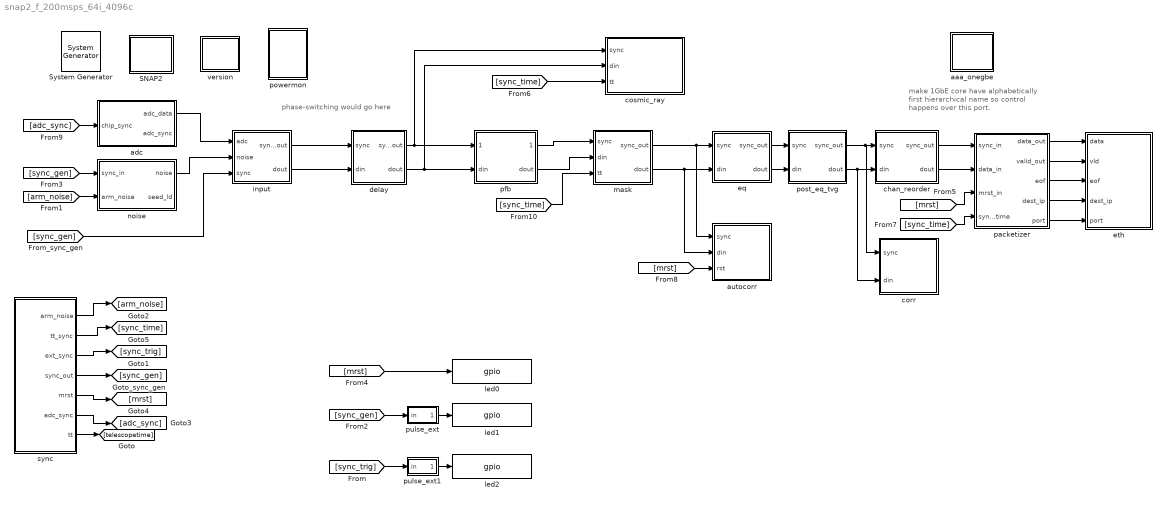
== system snap2_f_200msps_64i_4096c ==
  note: make 1GbE core have alphabetically
      | first hierarchical name so control
      | happens over this port.
  note: phase-switching
      | would go here
  " System Generator" : xbsIndex_r4/ System Generator  Tag=genX  xilinxfamily=kintexu  part=xcku115  speed=-2-e  package=flvf1924  synthesis_tool=XST  clock_wrapper=Clock Enables  directory=/home/jackh/src/caltech-lwa/snap2_f_200msps_64i_4096c/sysgen  proj_type=Vivado  Synth_file=Vivado Synthesis Defaults  Impl_file=Vivado Implementation Defaults  testbench=off  simulink_period=1  sysclk_period=5.102  dcm_input_clock_period=10  incr_netlist=off  trim_vbits=Everywhere in SubSystem  dbl_ovrd=According to Block Masks  core_generation=According to Block Masks  run_coregen=off  deprecated_control=off  eval_field=0  block_type=sysgen
  SNAP2 : Subsystem  Tag=xps:xsg  mask(xsg core config){hw_sys=SNAP2_v2:xcku115, clk_src=adc1_clk, clk_rate=196, use_microblaze=on, sample_period=1, synthesis_tool=XST}
      mask prompts: hw_sys "Hardware Platform"; clk_src "User IP Clock source"; clk_rate "User IP Clock Rate (MHz)"; use_microblaze "Use Microblaze controller?"; sample_period "Sample Period"; synthesis_tool "Synthesis Tool:"
      mask help:
      | The XSG Core Config block is used to configure the System Generator design
      | for the casper_xps toolflow. Settings here are used to configure the
      | Xilinx System Generator block parameters automatically, and control toolflow
      | script  execution. It needs to be at the top level of all designs being compiled
      | with the casper_xps toolflow.
      mask init:
      | xps_xsg_snap2_conf_mask;
      mask Help: eval('xlWeb([getenv(''MLIB_ROOT''), ''\doc\html\sys_xsg_core_config\sys_xsg_core_config.html''])')
      mask TypeOptions hw_sys: SNAP2_v1:xcku115 | SNAP2_v2:xcku115
      mask TypeOptions clk_src: sys_clk | clk_250MHz | adc0_clk | adc1_clk
      mask TypeOptions synthesis_tool: Leonardo Spectrum | Synplify | Synplify Pro | XST
      mask Display: fprintf(['SNAP2']);
  aaa_onegbe : Subsystem
  adc : Subsystem
  autocorr : Subsystem  mask{nchan_bits=12 - 3, npol_bits=6}
      mask prompts: nchan_bits "Number of *SERIAL* channels (2^?)"; npol_bits "Number of pols (2^?)"
  chan_reorder : Subsystem
  corr : Subsystem
  cosmic_ray : Subsystem
  delay : Subsystem  mask{max_delay_bits=12}
      mask prompts: max_delay_bits "Manimum delay (2^?) samples"
  eq : Subsystem
  eth : Subsystem
  input : Subsystem
  led0 : xps_library/IO/gpio  Tag=xps:gpio  io_group_params_forwarded=on  io_group=ROACH2:led  io_group_real=led  io_group_custom=0  io_dir=out  arith_type=Boolean  bitwidth=1  bin_pt=0  bit_index=0  sample_period=1  use_single_ended=off  use_ddr=off  reg_iob=on  reg_clk_phase=0  termination=None  use_iodelay=off
      settings: SourceProductName=CASPER XPS Blockset
  led1 : xps_library/IO/gpio  Tag=xps:gpio  io_group_params_forwarded=on  io_group=ROACH2:led  io_group_real=led  io_group_custom=0  io_dir=out  arith_type=Boolean  bitwidth=1  bin_pt=0  bit_index=1  sample_period=1  use_single_ended=off  use_ddr=off  reg_iob=on  reg_clk_phase=0  termination=None  use_iodelay=off
      settings: SourceProductName=CASPER XPS Blockset
  led2 : xps_library/IO/gpio  Tag=xps:gpio  io_group_params_forwarded=on  io_group=ROACH2:led  io_group_real=led  io_group_custom=0  io_dir=out  arith_type=Boolean  bitwidth=1  bin_pt=0  bit_index=2  sample_period=1  use_single_ended=off  use_ddr=off  reg_iob=on  reg_clk_phase=0  termination=None  use_iodelay=off
      settings: SourceProductName=CASPER XPS Blockset
  mask : Subsystem  mask{nfft_bits=12, ninput_bits=6}
      mask prompts: nfft_bits "FFT Channels (2^?)"; ninput_bits "Number of input signals (2^?)"
  noise : Subsystem
  packetizer : Subsystem  mask{nchan_bits=12, npol_bits=6, nparallel_bits=5}
      mask prompts: nchan_bits "Number of channels (including unsent) (2^?)"; npol_bits "Number of pols (2^?)"; nparallel_bits "Parallel samples (2^?)"
  pfb : Subsystem
  post_eq_tvg : Subsystem
  powermon : Subsystem
  pulse_ext : Subsystem  AncestorBlock=casper_library_misc/pulse_ext  mask(pulse_ext){pulse_len=2^26}
      mask prompts: pulse_len "Length of Pulse"
      mask help:
      | Extends a boolean signal to be high for the specified number of clocks after
      | the last high input.
      mask init:
      | bits = ceil(log2(pulse_len+1));
      mask Help: eval('xlWeb(''http://casper.berkeley.edu/wiki/Pulse_ext'')')
  pulse_ext1 : Subsystem  AncestorBlock=casper_library_misc/pulse_ext  mask(pulse_ext){pulse_len=2^26}
      mask prompts: pulse_len "Length of Pulse"
      mask help:
      | Extends a boolean signal to be high for the specified number of clocks after
      | the last high input.
      mask init:
      | bits = ceil(log2(pulse_len+1));
      mask Help: eval('xlWeb(''http://casper.berkeley.edu/wiki/Pulse_ext'')')
  sync : Subsystem  mask{sync_div_bits=30}
      mask prompts: sync_div_bits "Sync every 2^? FPGA clocks?"
  version : Subsystem  mask{ver_maj=7, ver_min=4, ver_rev=0, ver_bugfix=0}
      mask prompts: ver_maj "Major version"; ver_min "Minor version"; ver_rev "Revision"; ver_bugfix "Bugfix"
  wires:
  adc/1(adc_data) -> input/1(adc)
  noise/1(noise) -> input/2(noise)
  [arm_noise] -> noise/2(arm_noise)
  [sync_gen] -> noise/1(sync_in)
  [sync_gen] -> input/3(sync)
  post_eq_tvg/1(sync_out) -> corr/1(sync), chan_reorder/1(sync)
  post_eq_tvg/2(dout) -> chan_reorder/2(din), corr/2(din)
  [sync_gen] -> pulse_ext/1(in)
  [mrst] -> led0/1
  pulse_ext/1(out) -> led1/1
  [sync_trig] -> pulse_ext1/1(in)
  pulse_ext1/1(out) -> led2/1
  input/2(dout) -> delay/2(din)
  input/1(sync_out) -> delay/1(sync)
  chan_reorder/1(sync_out) -> packetizer/1(sync_in)
  chan_reorder/2(dout) -> packetizer/2(data_in)
  [mrst] -> packetizer/3(mrst_in)
  eq/1(sync_out) -> post_eq_tvg/1(sync)
  eq/2(dout) -> post_eq_tvg/2(din)
  sync/1(arm_noise) -> [arm_noise]
  sync/3(ext_sync) -> [sync_trig]
  sync/4(sync_out) -> [sync_gen]
  sync/2(tt_sync) -> [sync_time]
  sync/5(mrst) -> [mrst]
  [sync_time] -> packetizer/4(sync_time)
  packetizer/1(data_out) -> eth/1(data)
  packetizer/2(valid_out) -> eth/2(vld)
  packetizer/3(eof) -> eth/3(eof)
  packetizer/4(dest_ip) -> eth/4(dest_ip)
  packetizer/5(port) -> eth/5(port)
  [mrst] -> autocorr/3(rst)
  [adc_sync] -> adc/1(chip_sync)
  sync/6(adc_sync) -> [adc_sync]
  delay/1(sync_out) -> cosmic_ray/1(sync), pfb/1(sync_in)
  delay/2(dout) -> cosmic_ray/2(din), pfb/2(din)
  [sync_time] -> cosmic_ray/3(tt)
  sync/7(tt) -> [telescopetime]
  mask/1(sync_out) -> autocorr/1(sync), eq/1(sync)
  mask/2(dout) -> autocorr/2(din), eq/2(din)
  pfb/1(sync_out) -> mask/1(sync)
  pfb/2(dout) -> mask/2(din)
  [sync_time] -> mask/3(tt)
